simulink subsystem "kalmanFilter_V8SC"  (R2026a)
settings: Solver=VariableStepAuto
libraries: matrix_library x2
settings Model: Creator=lholliday  LastModifiedBy=lholliday

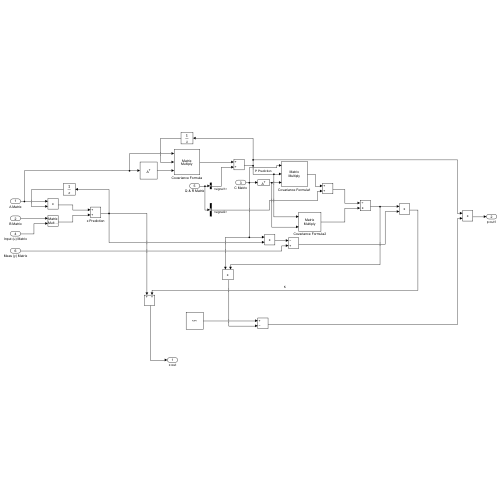
[thumbnail: Simulink's stored preview of the top-level diagram]
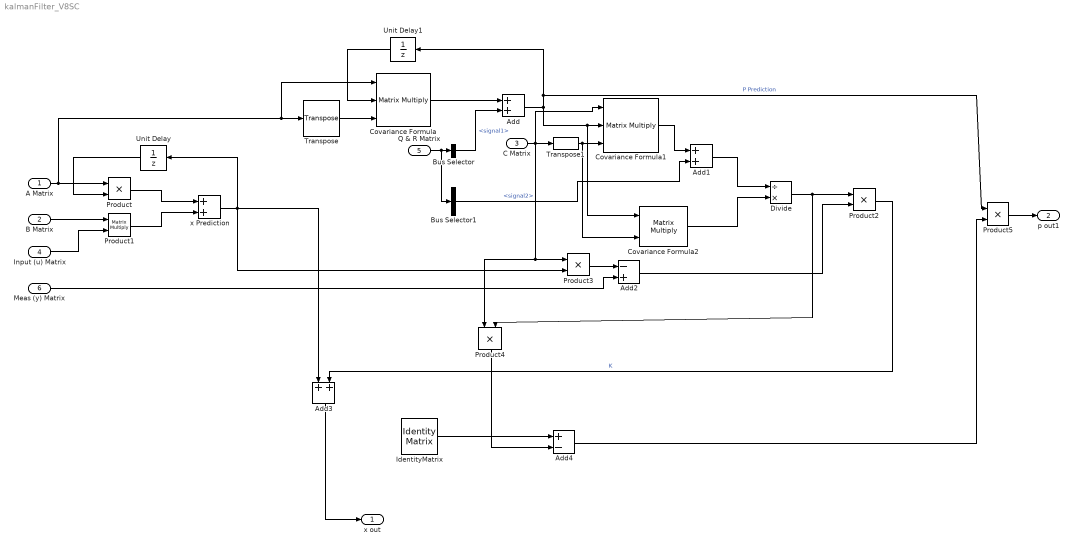
== system kalmanFilter_V8SC ==
  A Matrix : Inport
  B Matrix : Inport  Port=2
  C Matrix : Inport  Port=3
  Input (u) Matrix : Inport  Port=4
  Q & R Matrix : Inport  Port=5
  Meas (y) Matrix : Inport  Port=6
  Add : Sum
  Add1 : Sum
  Add2 : Sum  Inputs=-+
  Add3 : Sum
  Add4 : Sum  Inputs=+-
  Bus Selector : BusSelector  OutputSignals=signal1
  Bus Selector1 : BusSelector  OutputSignals=signal2
  Covariance Formula : Product  Inputs=3  Multiplication=Matrix(*)
  Covariance Formula1 : Product  Inputs=3  Multiplication=Matrix(*)
  Covariance Formula2 : Product  Multiplication=Matrix(*)
  Divide : Product  Inputs=/*
  IdentityMatrix : IdentityMatrix  OutputDimensions=4
  Product{,2..5} (5 alike) : Product
  Product1 : Product  Multiplication=Matrix(*)
  Transpose : matrix_library/Transpose
  Transpose1 : matrix_library/Transpose
  Unit Delay : UnitDelay  SampleTime=-1
  Unit Delay1 : UnitDelay  SampleTime=-1
  x Prediction : Sum
  x out : Outport
  p out1 : Outport  Port=2
  wires:
  A Matrix/1 -> Product/1, Covariance Formula/1, Transpose/1
  B Matrix/1 -> Product1/1
  Input (u) Matrix/1 -> Product1/2
  Product/1 -> x Prediction/1
  Product1/1 -> x Prediction/2
  x Prediction/1 -> Add3/1, Product3/2, Unit Delay/1
  Unit Delay/1 -> Product/2
  Transpose/1 -> Covariance Formula/3
  Covariance Formula/1 -> Add/1
  Unit Delay1/1 -> Covariance Formula/2
  Q & R Matrix/1 -> Bus Selector1/1, Bus Selector/1
  Bus Selector/1 -> Add/2  "<signal1>"
  Add/1 -> Product5/1, Unit Delay1/1, Covariance Formula2/1, Covariance Formula1/2  "P Prediction"
  Transpose1/1 -> Covariance Formula2/2, Covariance Formula1/3
  Bus Selector1/1 -> Add1/2  "<signal2>"
  Covariance Formula1/1 -> Add1/1
  Add1/1 -> Divide/1
  Covariance Formula2/1 -> Divide/2
  Divide/1 -> Product4/2, Product2/1
  Meas (y) Matrix/1 -> Add2/2
  Product3/1 -> Add2/1
  Add2/1 -> Product2/2
  Product2/1 -> Add3/2  "K"
  Add3/1 -> x out/1
  C Matrix/1 -> Product3/1, Product4/1, Transpose1/1, Covariance Formula1/1
  IdentityMatrix/1 -> Add4/1
  Product4/1 -> Add4/2
  Add4/1 -> Product5/2
  Product5/1 -> p out1/1
